simulink model "pos_id_step_simu"  (R2020b)
settings: Solver=VariableStepAuto  StartTime=0.0  StopTime=tfinal  RelTol=1e-3
values from neighbouring files (symbols this model uses):
  Kp_id = 0.2    [pos_id_step.m]
  r = 60    [pos_id_step.m]
  r_cyc = 8    [pos_id_step.m]
  ts = 1/50    (= 0.02)    [pos_id_step.m]
libraries: arduino_io_lib x5
settings Model: Creator=kei55  LastModifiedBy=kei55

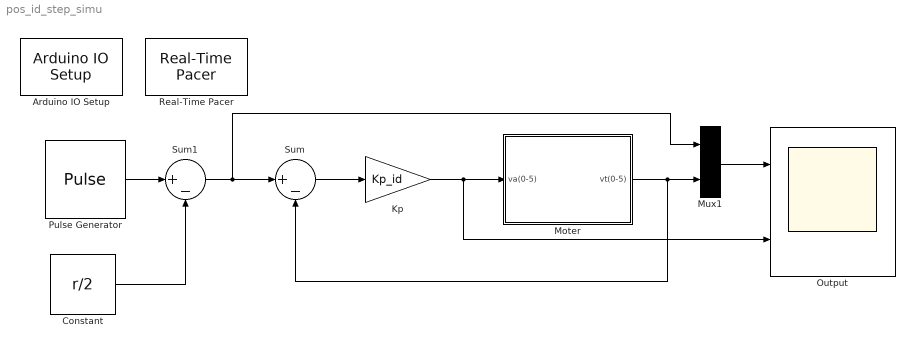
== system pos_id_step_simu ==
  Arduino IO Setup : arduino_io_lib/Arduino IO Setup  Priority=3  arduinoVar=Temporary arduino variable: Arduino1  workspaceVarName=a  comPort=COM3
  Constant : Constant  Value=r/2
  Kp : Gain  Gain=Kp_id
  Moter : Subsystem
  Mux1 : Mux  Inputs=2
  Output : Scope  NumInputPorts=2
  Pulse Generator : DiscretePulseGenerator  PulseType=Time based  Amplitude=r  Period=r_cyc  PulseWidth=50  SampleTime=1/50
  Real-Time Pacer : arduino_io_lib/Real-Time Pacer  simTimePerRealTime=1
  Sum : Sum  Inputs=|+-
  Sum1 : Sum  Inputs=|+-
  wires:
  Pulse Generator/1 -> Sum1/1
  Constant/1 -> Sum1/2
  Sum1/1 -> Mux1/1, Sum/1
  Moter/1(vt(0-5)) -> Sum/2, Mux1/2
  Sum/1 -> Kp/1
  Kp/1 -> Output/2, Moter/1(va(0-5))
  Mux1/1 -> Output/1

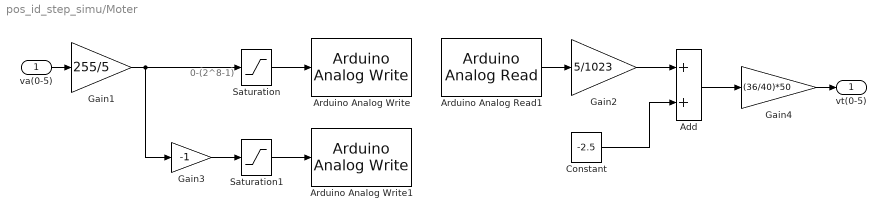
== system pos_id_step_simu/Moter ==
  note: 0-(2^8-1)
  va(0-5) : Inport
  Add : Sum
  Arduino Analog Read1 : arduino_io_lib/Arduino Analog Read  arduinoVar=Temporary arduino variable: Arduino1  arduinoPin=0  T=ts
  Arduino Analog Write : arduino_io_lib/Arduino Analog Write  arduinoVar=Temporary arduino variable: Arduino1  arduinoPin=3  T=ts
  Arduino Analog Write1 : arduino_io_lib/Arduino Analog Write  arduinoVar=Temporary arduino variable: Arduino1  arduinoPin=5  T=ts
  Constant : Constant  Value=-2.5
  Gain1 : Gain  Gain=255/5
  Gain2 : Gain  Gain=5/1023
  Gain3 : Gain  Gain=-1
  Gain4 : Gain  Gain=(36/40)*50
  Saturation : Saturate  UpperLimit=255  LowerLimit=0
  Saturation1 : Saturate  UpperLimit=255  LowerLimit=0
  vt(0-5) : Outport
  wires:
  Arduino Analog Read1/1 -> Gain2/1
  va(0-5)/1 -> Gain1/1
  Saturation/1 -> Arduino Analog Write/1
  Saturation1/1 -> Arduino Analog Write1/1
  Gain1/1 -> Gain3/1, Saturation/1
  Gain3/1 -> Saturation1/1
  Gain4/1 -> vt(0-5)/1
  Gain2/1 -> Add/1
  Constant/1 -> Add/2
  Add/1 -> Gain4/1
